simulink model "psopid"  (R2019a)
settings: Solver=VariableStepAuto  StartTime=0.0  StopTime=Temp  RelTol=1e-3
values from neighbouring files (symbols this model uses):
  den = [1 17 80 100]    [PID_verification.m]
  gama = 1/8    (= 0.125)    [PID_verification.m]
  Kp = 0.49364697362150595    (= 0.493646973622)    [PID_verification.m]
  num = [200 1200]    [PID_verification.m]
  Td = 0.07822875867824934;v    [PID_verification.m]
  Ti = 0.655067793547871    (= 0.655067793548)    [PID_verification.m]
undefined symbols (not defined in the file or in its folder): magnitude
settings Model: Creator=vitor  LastModifiedBy=vitor

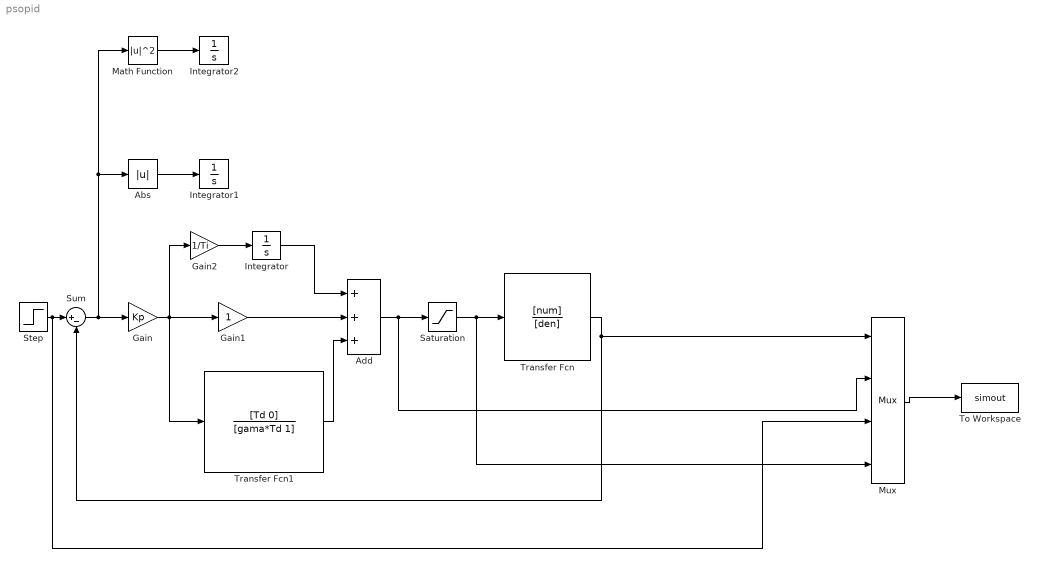
== system psopid ==
  Abs : Abs
  Add : Sum  Inputs=+++
  Gain : Gain  Gain=Kp
  Gain1 : Gain
  Gain2 : Gain  Gain=1/Ti
  Integrator : Integrator
  Integrator1 : Integrator
  Integrator2 : Integrator
  Math Function : Math  Operator=magnitude^2  SaturateOnIntegerOverflow=on
  Mux : Mux
  Saturation : Saturate  UpperLimit=100  LowerLimit=0
  Step : Step  SampleTime=0
  Sum : Sum  Inputs=|+-
  To Workspace : ToWorkspace  VariableName=simout  SampleTime=-1
  Transfer Fcn : TransferFcn  Numerator=[num]  Denominator=[den]
  Transfer Fcn1 : TransferFcn  Numerator=[Td 0]  Denominator=[gama*Td 1]
  wires:
  Sum/1 -> Math Function/1, Abs/1, Gain/1
  Gain/1 -> Gain2/1, Transfer Fcn1/1, Gain1/1
  Gain1/1 -> Add/2
  Gain2/1 -> Integrator/1
  Transfer Fcn1/1 -> Add/3
  Integrator/1 -> Add/1
  Add/1 -> Mux/2, Saturation/1
  Transfer Fcn/1 -> Mux/1, Sum/2
  Mux/1 -> To Workspace/1
  Saturation/1 -> Mux/4, Transfer Fcn/1
  Step/1 -> Mux/3, Sum/1
  Abs/1 -> Integrator1/1
  Math Function/1 -> Integrator2/1
